simulink model "failureInputReadF16"  (R2024a)
settings: configuration reference "standardSILConfiguraitonParams" (kept outside this file)
undefined symbols (not defined in the file): EnumF16FailureType
libraries: simulink x5
settings Model: Creator=jerem  LastModifiedBy=jerem
settings ConfigSetRef: SourceName=standardSILConfiguraitonParams  SourceLocation=Base Workspace

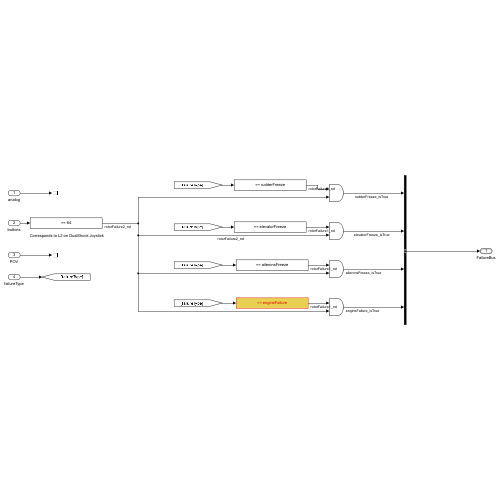
[thumbnail: Simulink's stored preview of the top-level diagram]
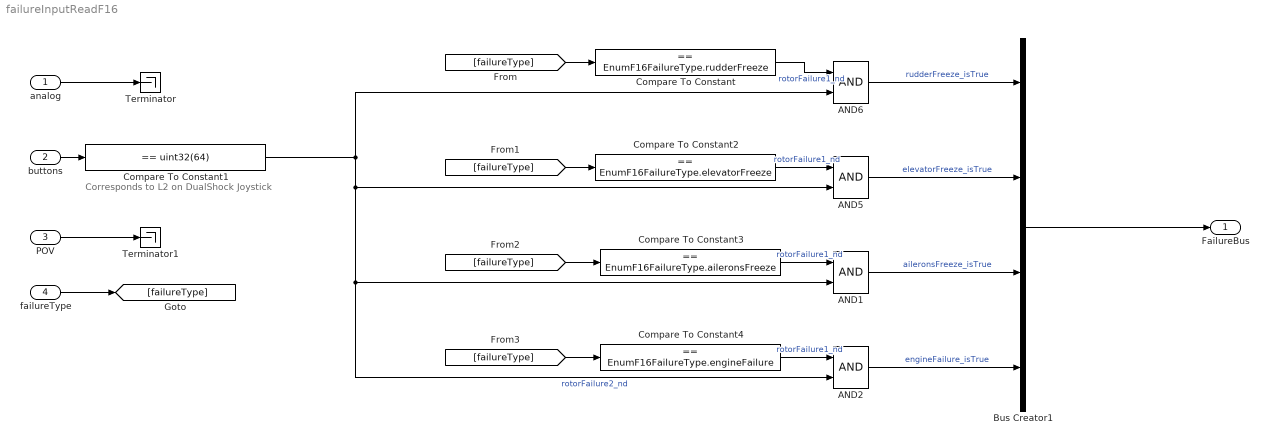
== system failureInputReadF16 ==
  note: Corresponds to L2 on DualShock Joystick
  analog : Inport  PortDimensions=6
  buttons : Inport  Port=2  OutDataTypeStr=uint32
  POV : Inport  Port=3
  failureType : Inport  Port=4  OutDataTypeStr=Enum:EnumF16FailureType
  AND{1..2,5..6} (4 alike) : Logic  IconShape=distinctive  AllPortsSameDT=off  OutDataTypeStr=boolean
  Bus Creator1 : BusCreator  Inputs=4  OutDataTypeStr=Bus: FailureBus
  Compare To Constant : simulink/Logic and Bit Operations/Compare To Constant  relop===  const=EnumF16FailureType.rudderFreeze  OutDataTypeStr=boolean
  Compare To Constant1 : simulink/Logic and Bit Operations/Compare To Constant  relop===  const=uint32(64)  OutDataTypeStr=boolean
  Compare To Constant2 : simulink/Logic and Bit Operations/Compare To Constant  relop===  const=EnumF16FailureType.elevatorFreeze  OutDataTypeStr=boolean
  Compare To Constant3 : simulink/Logic and Bit Operations/Compare To Constant  relop===  const=EnumF16FailureType.aileronsFreeze  OutDataTypeStr=boolean
  Compare To Constant4 : simulink/Logic and Bit Operations/Compare To Constant  relop===  const=EnumF16FailureType.engineFailure  OutDataTypeStr=boolean
  Terminator : Terminator
  Terminator1 : Terminator
  FailureBus : Outport  OutDataTypeStr=Bus: FailureBus
  wires:
  analog/1 -> Terminator/1
  Compare To Constant3/1 -> AND1/1  "rotorFailure1_nd"
  failureType/1 -> [failureType]
  Compare To Constant/1 -> AND6/1  "rotorFailure1_nd"
  AND1/1 -> Bus Creator1/3  "aileronsFreeze_isTrue"
  AND6/1 -> Bus Creator1/1  "rudderFreeze_isTrue"
  [failureType] -> Compare To Constant3/1
  Bus Creator1/1 -> FailureBus/1
  POV/1 -> Terminator1/1
  AND5/1 -> Bus Creator1/2  "elevatorFreeze_isTrue"
  buttons/1 -> Compare To Constant1/1
  [failureType] -> Compare To Constant/1
  Compare To Constant2/1 -> AND5/1  "rotorFailure1_nd"
  [failureType] -> Compare To Constant2/1
  Compare To Constant1/1 -> AND5/2, AND2/2, AND1/2, AND6/2  "rotorFailure2_nd"
  Compare To Constant4/1 -> AND2/1  "rotorFailure1_nd"
  [failureType] -> Compare To Constant4/1
  AND2/1 -> Bus Creator1/4  "engineFailure_isTrue"
